simulink model "PD_planar_3R"  (R2020b)
settings: Solver=ode8  StartTime=0.0  StopTime=T  FixedStep=0.001  RelTol=1e-3
values from neighbouring files (symbols this model uses):
  F = 1000*[-sin(q0(1)+q0(2)+q0(3)); cos(q0(1)+q0(2)+q0(3))]    [main.m]    (also in main_linear.m)
  fpi_params = [eta0 eps max_it]    [main.m]
  invB = B^-1    [main.m]    (also in main_linear.m = inv(B))
  Kd = diag([500 500 500])    [main.m]    (also in main_linear.m = diag([kd_par kd_par kd_par]))
  Kp = diag([800 800 800])    [main.m]    (also in main_linear.m = diag([kp_par kp_par kp_par]))
  link = 1    [main.m]    (also in main_linear.m = 3)
  motor = [I_m*k_r^2,k]    [main.m]    (also in main_linear.m = [I_m*k_r^2, k, k_new])
  param = [m mm d I g0]'    [main.m]    (also in main_linear.m)
  q0 = qd    [main.m]    (also in main_linear.m)
  qd = [pi/3; -pi/4; pi/3]    [main.m]    (also in main_linear.m = [pi/3; -pi/7; pi/4])
  qd0 = [0;0;0]    [main.m]    (also in main_linear.m = [0; 0; 0])
  T1 = 5    [main.m]    (also in main_linear.m = 2)
  T2 = 5.5    [main.m]    (also in main_linear.m = 3)
  theta0 = q0    [main.m]    (also in main_linear.m)
  thetad0 = [0;0;0]    [main.m]    (also in main_linear.m = [0; 0; 0])
settings Model: Creator=lorenzo  LastModifiedBy=lorenzo

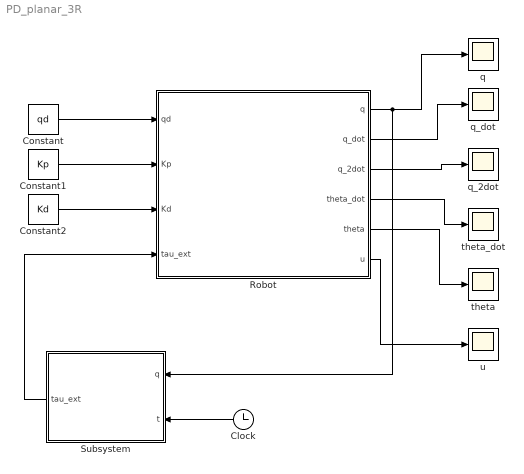
== system PD_planar_3R ==
  Clock : Clock
  Constant : Constant  Value=qd  VectorParams1D=off
  Constant1 : Constant  Value=Kp  VectorParams1D=off
  Constant2 : Constant  Value=Kd  VectorParams1D=off
  Robot : Subsystem
  Subsystem : Subsystem
  q : Scope
  q_2dot : Scope
  q_dot : Scope
  theta : Scope
  theta_dot : Scope
  u : Scope
  wires:
  Constant/1 -> Robot/1(qd)
  Constant1/1 -> Robot/2(Kp)
  Constant2/1 -> Robot/3(Kd)
  Robot/2(q_dot) -> q_dot/1
  Robot/3(q_2dot) -> q_2dot/1
  Robot/4("theta_dot ") -> theta_dot/1
  Robot/5(theta) -> theta/1
  Robot/6(u) -> u/1
  Robot/1(q) -> Subsystem/1(q), q/1
  Clock/1 -> Subsystem/2(t)
  Subsystem/1(tau_ext) -> Robot/4(tau_ext)

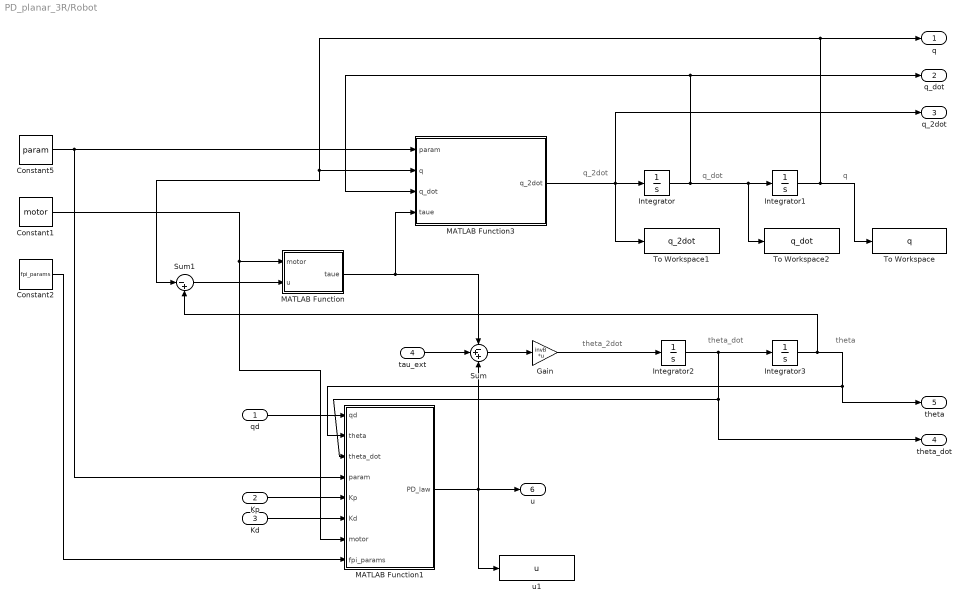
== system PD_planar_3R/Robot ==
  note: theta_2dot
  note: q_dot
  note: theta_dot
  note: q
  note: q_2dot
  note: theta
  qd : Inport
  Kp : Inport  Port=2
  Kd : Inport  Port=3
  tau_ext : Inport  Port=4
  Constant1 : Constant  Value=motor  VectorParams1D=off
  Constant2 : Constant  Value=fpi_params  VectorParams1D=off
  Constant5 : Constant  Value=param  VectorParams1D=off
  Gain : Gain  Gain=invB  Multiplication=Matrix(K*u) (u vector)
  Integrator : Integrator  InitialCondition=qd0
  Integrator1 : Integrator  InitialCondition=q0
  Integrator2 : Integrator  InitialCondition=thetad0
  Integrator3 : Integrator  InitialCondition=theta0
  MATLAB Function : MATLAB Function  TreatAsAtomicUnit=on
  MATLAB Function1 : MATLAB Function  TreatAsAtomicUnit=on
  MATLAB Function3 : MATLAB Function  TreatAsAtomicUnit=on
  Sum : Sum  Inputs=-++
  Sum1 : Sum  Inputs=|-+
  To Workspace : ToWorkspace  VariableName=q  SampleTime=-1
  To Workspace1 : ToWorkspace  VariableName=q_2dot  SampleTime=-1
  To Workspace2 : ToWorkspace  VariableName=q_dot  SampleTime=-1
  u1 : ToWorkspace  VariableName=u  SampleTime=-1
  q : Outport
  q_dot : Outport  Port=2
  q_2dot : Outport  Port=3
  "theta_dot " : Outport  Port=4
  theta : Outport  Port=5
  u : Outport  Port=6
  wires:
  Sum1/1 -> MATLAB Function/2(u)
  Integrator2/1 -> MATLAB Function1/3(theta_dot), "theta_dot "/1, Integrator3/1
  MATLAB Function3/1(q_2dot) -> To Workspace1/1, q_2dot/1, Integrator/1
  Constant5/1 -> MATLAB Function3/1(param), MATLAB Function1/4(param)
  MATLAB Function/1(taue) -> MATLAB Function3/4(taue), Sum/1
  Sum/1 -> Gain/1
  Integrator3/1 -> MATLAB Function1/2(theta), theta/1, Sum1/2
  Integrator1/1 -> Sum1/1, MATLAB Function3/2(q), q/1, To Workspace/1
  Gain/1 -> Integrator2/1
  Integrator/1 -> q_dot/1, MATLAB Function3/3(q_dot), To Workspace2/1, Integrator1/1
  Constant1/1 -> MATLAB Function1/7(motor), MATLAB Function/1(motor)
  MATLAB Function1/1(PD_law) -> u1/1, u/1, Sum/3
  qd/1 -> MATLAB Function1/1(qd)
  Kp/1 -> MATLAB Function1/5(Kp)
  Kd/1 -> MATLAB Function1/6(Kd)
  Constant2/1 -> MATLAB Function1/8(fpi_params)
  tau_ext/1 -> Sum/2

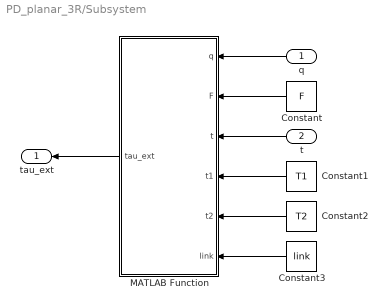
== system PD_planar_3R/Subsystem ==
  q : Inport
  t : Inport  Port=2
  Constant : Constant  Value=F  VectorParams1D=off
  Constant1 : Constant  Value=T1  VectorParams1D=off
  Constant2 : Constant  Value=T2  VectorParams1D=off
  Constant3 : Constant  Value=link  VectorParams1D=off
  MATLAB Function : MATLAB Function  TreatAsAtomicUnit=on
  tau_ext : Outport
  wires:
  q/1 -> MATLAB Function/1(q)
  t/1 -> MATLAB Function/3(t)
  Constant1/1 -> MATLAB Function/4(t1)
  MATLAB Function/1(tau_ext) -> tau_ext/1
  Constant2/1 -> MATLAB Function/5(t2)
  Constant3/1 -> MATLAB Function/6(link)
  Constant/1 -> MATLAB Function/2(F)

== matlab function PD_planar_3R/Robot/MATLAB Function1 ==
  data: qd input; theta input; theta_dot input; PD_law output; param input; Kp input; Kd input; motor input; fpi_params input
function PD_law = fcn(qd, theta, theta_dot, param, Kp, Kd, motor, fpi_params)

q1 = qd(1);
q2 = qd(2);
q3 = qd(3);

% masses of the links
m1 = param(1);
m2 = m1;
m3 = m1;

% masses of the motors
m1m = param(2);
m2m = m1m;
m3m = m1m;

% distance from the CoMs
d1 = param(3);
d2 = d1;
d3 = d1;

% inertia of the links
I1 = param(4);
I2 = I1;
I3 = I1;

% acceleration of gravity
g0 = param(5);


%% Gravity term

l1 = 1;
l2 = 1;

g = [g0*m2*(d2*cos(q1 + q2) + l1*cos(q1)) + g0*m3*(l2*cos(q1 + q2) + d3*cos(q1 + q2 + q3) + l1*cos(q1)) + d1*g0*m1*cos(q1);
                                                g0*m3*(l2*cos(q1 + q2) + d3*cos(q1 + q2 + q3)) + d2*g0*m2*cos(q1 + q2);
                                                                                            d3*g0*m3*cos(q1 + q2 + q3)];

g_d = [g0*m2*(d2*cos(qd(1) + qd(2)) + l1*cos(qd(1))) + g0*m3*(l2*cos(qd(1) + qd(2)) + d3*cos(qd(1) + qd(2) + qd(3)) + l1*cos(qd(1))) + d1*g0*m1*cos(qd(1));
                                                g0*m3*(l2*cos(qd(1) + qd(2)) + d3*cos(qd(1) + qd(2) + qd(3))) + d2*g0*m2*cos(qd(1) + qd(2));
                                                                                            d3*g0*m3*cos(qd(1) + qd(2) + qd(3))];
%% Stiffness matrix

k = motor(2);
K = k*eye(3);
invK = inv(K);

%% Desired theta

%theta_d = qd + invK*g;

% initialize the algorithm
theta_d = zeros(3, 1);

theta0 = fpi_params(1);
eps = fpi_params(2);
max_it = fpi_params(3);

for i = 1:3
    
    % initial guess
    theta_temp = theta0;
    
    % initialization of variables for the while loop
    j = 1;
    fun = 2*eps;
    
    % stops if we reach the maximum number of iteration or if we have a
    % sufficiently small error
    while (j < max_it) && (fun > eps)
        
        % error between function evaluated in the guess and the real value
        fun = -sin(theta_temp - qd(i)) + 1/k*g_d(i);
        
        % update theta value
        theta_temp = theta_temp + fun;
        
        % true error
        fun = abs(fun);
        
        j = j + 1;
    end
    
    % assign the vaue of eta
    theta_d(i) = theta_temp;
    
end




%% Control law

PD_law = -Kp*(theta-theta_d)-Kd*theta_dot+g;

== matlab function PD_planar_3R/Robot/MATLAB Function3 ==
  data: param input; q input; q_2dot output size=[3 1]; q_dot input; taue input
function q_2dot = q_2dot(param, q, q_dot, taue)
%% Initialization of the variables

q1 = q(1);
q2 = q(2);
q3 = q(3);

q1d = q_dot(1);
q2d = q_dot(2);
q3d = q_dot(3);

% masses of the links
m1 = param(1);
m2 = m1;
m3 = m1;

% masses of the motors
m1m = param(2);
m2m = m1m;
m3m = m1m;

% distance from the CoMs
d1 = param(3);
d2 = d1;
d3 = d1;

% inertia of the links
I1 = param(4);
I2 = I1;
I3 = I1;

% acceleration of gravity
g0 = param(5);

a1 = m3*d3^2+I3;
a2 = m3*d3;
a3 = d3*m3;
a4 = I2+I3+d2^2*m2+d3^2*m3+m3+m3m;
a5 = m2*d2+m3m+m3;
a6 = I1+I2+I3+d1^2*m1+d2^2*m2+d3^2*m3+m1+m3+m3+m2m+m3m+m3m;

%% Inertia matrix

m11 = a6+2*a3*cos(q2+q3)+2*a5*cos(q2)+2*a2*cos(q3);
m12 = a4+a3*cos(q2+q3)+2*a2*cos(q3)+a5*cos(q2);
m13 = a1+a2*cos(q3)+a3*cos(q2+q3);
m21 = m12;
m22 = a4+2*a2*cos(q3);
m23 = a1+a2*cos(q3);
m31 = m13;
m32 = m23;
m33 = a1;

M = [m11 m12 m13;
    m21 m22 m23;
    m31 m32 m33];

%% Coriolis term

C = [- a3*q2d^2*sin(q2 + q3) - a3*q3d^2*sin(q2 + q3) - a2*q3d^2*sin(q3) - a5*q2d^2*sin(q2) - 2*a3*q1d*q2d*sin(q2 + q3) - 2*a3*q1d*q3d*sin(q2 + q3) - 2*a3*q2d*q3d*sin(q2 + q3) - 2*a2*q1d*q3d*sin(q3) - 2*a2*q2d*q3d*sin(q3) - 2*a5*q1d*q2d*sin(q2);
                                                                                                                                      a3*q1d^2*sin(q2 + q3) - a2*q3d^2*sin(q3) + a5*q1d^2*sin(q2) - 2*a2*q1d*q3d*sin(q3) - 2*a2*q2d*q3d*sin(q3);
                                                                                                                                                             a3*q1d^2*sin(q2 + q3) + a2*q1d^2*sin(q3) + a2*q2d^2*sin(q3) + 2*a2*q1d*q2d*sin(q3)];

%% Gravity term

l1 = 1;
l2 = 1;

g = [g0*m2*(d2*cos(q1 + q2) + l1*cos(q1)) + g0*m3*(l2*cos(q1 + q2) + d3*cos(q1 + q2 + q3) + l1*cos(q1)) + d1*g0*m1*cos(q1);
                                                g0*m3*(l2*cos(q1 + q2) + d3*cos(q1 + q2 + q3)) + d2*g0*m2*cos(q1 + q2);
                                                                                            d3*g0*m3*cos(q1 + q2 + q3)];


%% q_2dot

q_2dot = M^-1*(taue-C-g);

== matlab function PD_planar_3R/Robot/MATLAB Function ==
  data: motor input; u input; taue output
function taue = fcn(motor, u)

k = motor(2);

taue = [k*sin(u(1)); k*sin(u(2)); k*sin(u(3))];
%taue = [k*u(1); k*u(2); k*u(3)];

== matlab function PD_planar_3R/Subsystem/MATLAB Function ==
  data: q input; tau_ext output; F input; t input; t1 input; t2 input; link input
function tau_ext = tau_ext(q, F, t, t1, t2, link)

tau_ext = zeros(3,1);

s1 = sin(q(1));
s12 = sin(q(1)+q(2));
s123 = sin(q(1)+q(2)+q(3));
c1 = cos(q(1));
c12 = cos(q(1)+q(2));
c123 = cos(q(1)+q(2)+q(3));
J = zeros(2, 3);

% choose the particular jacobian coordingly to where the external force
% acts
switch link
    case 1
        J = 0.5*[-s1 0 0; c1 0 0];
    case 2
        J = 0.5*[-s1-s12 -s12 0; c1+c12 c12 0];
    case 3
        J = 0.5*[-s1-s12-s123 -s12-s123 -s123; c1+c12+c123 c12+c123 c123];
end

if t>=t1 && t<=t2
    tau_ext = -J'*F;
end
